simulink model "simulation_quad_modif_nu"  (R2020b)
settings: Solver=VariableStepAuto  StartTime=0.0  StopTime=30  RelTol=1e-3
values from neighbouring files (symbols this model uses):
  controlleur = struct('kap',2.0,                       'kad',4.0,                       'kpp',4.0,                       'kpd',8.0,                       'k_delta',15.0,                       'u_barre',u_barre,                       'M_k',M_k,                       'skew_sym_d_etoile',skew_sym_d_etoile,                       'd_etoile', d_etoile                       )    [generateContolleur.m]    (also in run_quad.m = generateContolleur(drone))
  drone = generatequad()    [run_quad.m]
  f_initial = 1    [run_quad.m]
  initial_state = [p_initial; v_initial; omega_initial; q_initial]    [run_quad.m]
  position_cible = 0.5*[1; 1; 1]    [run_quad.m]
  q_d_initial = ToQuaternion(yaw_d, pitch_d, roll_d)    [run_quad.m]
settings Model: Creator=florian  LastModifiedBy=florian

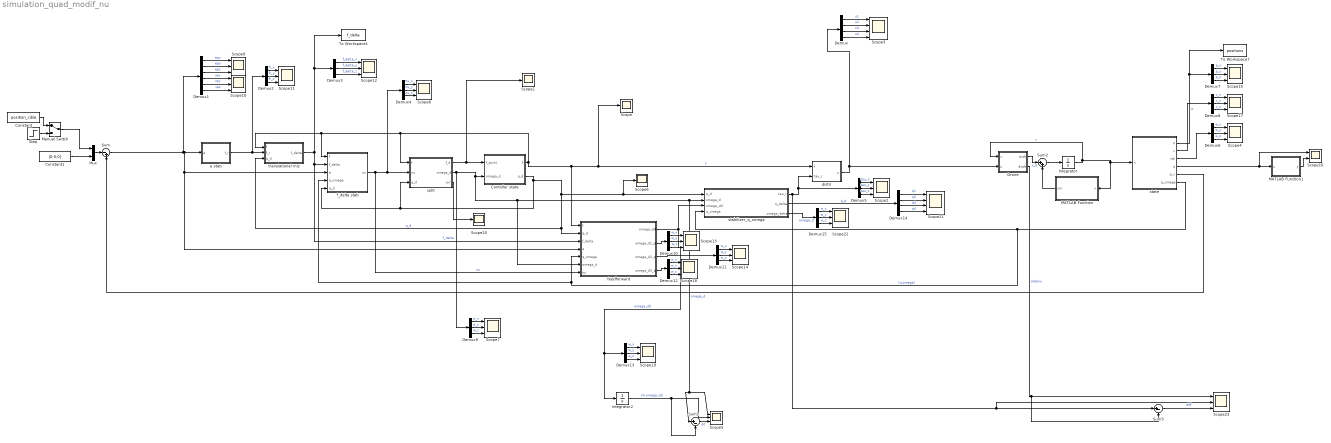
== system simulation_quad_modif_nu ==
  Constant : Constant  Value=position_cible
  Constant1 : Constant  Value=[0;0;0]
  Contoller state : Subsystem
  Demux : Demux
  Demux1 : Demux  Outputs=6
  Demux{2..13,15} (13 alike) : Demux  Outputs=3
  Demux14 : Demux
  Drone : MATLAB Function  TreatAsAtomicUnit=on
  Integrator : Integrator  InitialCondition=initial_state
  Integrator2 : Integrator
  MATLAB Function : MATLAB Function  TreatAsAtomicUnit=on
  MATLAB Function1 : MATLAB Function  TreatAsAtomicUnit=on
  Manual Switch : ManualSwitch
  Mux : Mux  Inputs=2
  Scope{,1,6,20} (4 alike) : Scope
  Scope{2,4..5,7..15,17..19,22..23} (17 alike) : Scope  NumInputPorts=3
  Scope16 : Scope  NumInputPorts=2
  Scope21 : Scope  NumInputPorts=4
  Scope3 : Scope  NumInputPorts=4
  Step : Step  Time=10  Before=position_cible  After=[0;0;0]  SampleTime=0
  Sum : Sum  Inputs=|-+
  Sum1 : Sum  Inputs=|+-
  Sum2 : Sum  Inputs=|++
  Sum3 : Sum  Inputs=|+-
  To Workspace1 : ToWorkspace  VariableName=f_delta  SampleTime=-1
  To Workspace7 : ToWorkspace  VariableName=positions  SampleTime=-1
  distri : MATLAB Function  TreatAsAtomicUnit=on
  e stab : MATLAB Function  TreatAsAtomicUnit=on
  f_delta stab : MATLAB Function  TreatAsAtomicUnit=on
  feedforward : MATLAB Function  TreatAsAtomicUnit=on
  split : MATLAB Function  TreatAsAtomicUnit=on
  stabilizer_q_omega : MATLAB Function  TreatAsAtomicUnit=on
  state : MATLAB Function  TreatAsAtomicUnit=on
  translational mis : MATLAB Function  TreatAsAtomicUnit=on
  wires:
  Integrator/1 -> Drone/1(x), MATLAB Function/1(x), state/1(x)  "x"
  Demux7/2 -> Scope15/2  "p_y"
  state/1(p) -> To Workspace7/1, Demux7/1  "p"
  state/4(q) -> Scope16/1, MATLAB Function1/1(u)
  Demux8/3 -> Scope17/3  "v_z"
  Demux8/1 -> Scope17/1  "v_x"
  MATLAB Function1/1(y) -> Scope16/2
  Demux8/2 -> Scope17/2  "v_y"
  state/2(v) -> Demux8/1
  Demux7/1 -> Scope15/1  "p_x"
  Demux7/3 -> Scope15/3  "p_z"
  Drone/1(dxdt) -> Sum2/1  "x_d"
  Sum2/1 -> Integrator/1
  MATLAB Function/1(cor) -> Sum2/2
  Demux6/2 -> Scope4/2  "w_y"
  Demux6/3 -> Scope4/3  "w_z"
  state/3(wb) -> Demux6/1
  Demux6/1 -> Scope4/1  "w_x"
  Constant1/1 -> Mux/2
  Demux4/2 -> Scope8/2  "nu_y"
  f_delta stab/1(nu) -> feedforward/7(nu), Demux4/1, split/2(nu)  "nu"
  Demux9/1 -> Scope7/1  "w_x"
  Mux/1 -> Sum/1
  split/3(err) -> Scope20/1
  Step/1 -> Manual Switch/2
  Constant/1 -> Manual Switch/1
  Demux11/2 -> Scope14/2  "w_y"
  Contoller state/1(f) -> f_delta stab/1(f), translational mis/1(f), split/1(f), feedforward/1(f), Scope/1, distri/1(f)  "f"
  feedforward/1(omega_dd) -> stabilizer_q_omega/3(omega_dd), Demux13/1, Integrator2/1  "omega_dd"
  Demux13/2 -> Scope19/2  "w_y"
  Demux3/1 -> Scope12/1  "f_delta_x"
  Demux1/4 -> Scope10/1  "vpx"
  Demux/2 -> Scope3/2  "u2"
  Demux9/3 -> Scope7/3  "w_z"
  state/6(q_omega) -> f_delta stab/4(q_omega), feedforward/5(q_omega), stabilizer_q_omega/4(q_omega)  "(q,omega)"
  Demux12/2 -> Scope18/2  "w_y"
  state/5(p_v) -> Sum/2
  Demux3/3 -> Scope12/3  "f_delta_z"
  Manual Switch/1 -> Mux/1
  Demux13/1 -> Scope19/1  "w_x"
  Demux11/3 -> Scope14/3  "w_z"
  Demux/4 -> Scope3/4  "u4"
  Demux2/1 -> Scope11/1  "fr_x"
  Demux13/3 -> Scope19/3  "w_z"
  Demux10/3 -> Scope13/3  "w_z"
  Demux9/2 -> Scope7/2  "w_y"
  Demux5/2 -> Scope2/2  "tau_y"
  e stab/1(f_r) -> Demux2/1, translational mis/2(f_r)
  Demux/1 -> Scope3/1  "u1"
  Demux2/2 -> Scope11/2  "fr_y"
  feedforward/3(omega_d2_p) -> Demux11/1
  Demux15/3 -> Scope22/3  "w_z"
  Demux4/3 -> Scope8/3  "nu_z"
  Demux14/4 -> Scope21/4  "q4"
  split/2(omega_d) -> Demux9/1, feedforward/6(omega_d), Sum1/1, Scope5/1, stabilizer_q_omega/2(omega_d), Contoller state/2(omega_d)  "omega_d"
  Demux4/1 -> Scope8/1  "nu_x"
  Demux14/1 -> Scope21/1  "q1"
  Demux15/2 -> Scope22/2  "w_y"
  Contoller state/2(q_d) -> f_delta stab/5(q_d), split/3(q_d), feedforward/2(q_d), translational mis/3(q_d), Scope6/1, stabilizer_q_omega/1(q_d)  "q_d"
  feedforward/2(omega_d1_p) -> Demux10/1
  Demux15/1 -> Scope22/1  "w_x"
  stabilizer_q_omega/2(q_delta) -> Demux14/1  "q_d"
  Sum1/1 -> Scope5/3  "dif"
  Demux11/1 -> Scope14/1  "w_x"
  Demux12/1 -> Scope18/1  "w_x"
  Demux12/3 -> Scope18/3  "w_z"
  feedforward/4(omega_d3_p) -> Demux12/1
  Demux10/2 -> Scope13/2  "w_y"
  Demux1/2 -> Scope9/2  "epy"
  Demux10/1 -> Scope13/1  "w_x"
  distri/1(u) -> Drone/2(u), Demux/1
  Demux5/1 -> Scope2/1  "tau_x"
  Demux1/6 -> Scope10/3  "vpz"
  split/1(f_d) -> Scope1/1, Contoller state/1(f_point)
  Demux5/3 -> Scope2/3  "tau_z"
  Demux2/3 -> Scope11/3  "fr_z"
  Demux3/2 -> Scope12/2  "f_delta_y"
  stabilizer_q_omega/3(omega_delta) -> Demux15/1  "omega_d"
  Sum/1 -> Demux1/1, feedforward/4(e), f_delta stab/3(e), e stab/1(e)
  translational mis/1(f_delta) -> Demux3/1, To Workspace1/1, feedforward/3(f_delta), f_delta stab/2(f_delta)  "f_delta"
  Demux14/3 -> Scope21/3  "q3"
  Demux1/1 -> Scope9/1  "epx"
  Demux1/3 -> Scope9/3  "epz"
  Demux1/5 -> Scope10/2  "vpy"
  Demux/3 -> Scope3/3  "u3"
  Integrator2/1 -> Sum1/2, Scope5/2  "int omega_dd"
  Demux14/2 -> Scope21/2  "q2"
  Drone/2(dwdt) -> Sum3/2, Scope23/1  "obtenu"
  Sum3/1 -> Scope23/3  "diff"
  stabilizer_q_omega/1(tau_r) -> Scope23/2, Sum3/1, Demux5/1, distri/2(tau_r)

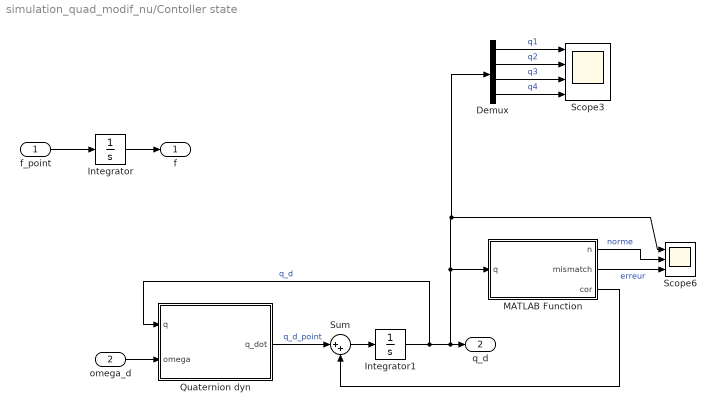
== system simulation_quad_modif_nu/Contoller state ==
  f_point : Inport
  omega_d : Inport  Port=2
  Demux : Demux
  Integrator : Integrator  InitialCondition=f_initial
  Integrator1 : Integrator  InitialCondition=q_d_initial
  MATLAB Function : MATLAB Function  TreatAsAtomicUnit=on
  Quaternion dyn : MATLAB Function  TreatAsAtomicUnit=on
  Scope3 : Scope  NumInputPorts=4
  Scope6 : Scope  NumInputPorts=3
  Sum : Sum  Inputs=|++
  f : Outport
  q_d : Outport  Port=2
  wires:
  Integrator/1 -> f/1
  f_point/1 -> Integrator/1
  Integrator1/1 -> Quaternion dyn/1(q), Demux/1, Scope6/1, MATLAB Function/1(q), q_d/1  "q_d"
  omega_d/1 -> Quaternion dyn/2(omega)
  Quaternion dyn/1(q_dot) -> Sum/1  "q_d_point"
  Sum/1 -> Integrator1/1
  MATLAB Function/3(cor) -> Sum/2
  MATLAB Function/1(n) -> Scope6/2  "norme"
  MATLAB Function/2(mismatch) -> Scope6/3  "erreur"
  Demux/3 -> Scope3/3  "q3"
  Demux/2 -> Scope3/2  "q2"
  Demux/1 -> Scope3/1  "q1"
  Demux/4 -> Scope3/4  "q4"

== matlab function simulation_quad_modif_nu/Contoller state/MATLAB Function ==
  data: n output; q input; mismatch output; cor output
function [n, mismatch, cor] = fcn(q)
%#codegen
n = norm(q);
mismatch = 1-norm(q);
cor = mismatch*q;

== matlab function simulation_quad_modif_nu/MATLAB Function1 ==
  data: u input; y output
function y = fcn(u)
%#codegen

y = norm(u);

== matlab function simulation_quad_modif_nu/Contoller state/Quaternion dyn ==
  data: q input; q_dot output; omega input
function q_dot = q_dyn(q, omega)
%#codegen

eta = q(1);
eps = q(2:4);

A = [-eps';  eta*eye(3)+skew_sym(eps)];
q_dot = 1/2*A*omega;

== matlab function simulation_quad_modif_nu/state ==
  data: x input; p output; v output; wb output; q output; p_v output; q_omega output
function [p, v, wb, q, p_v, q_omega] = demux(x)
%#codegen

p = x(1:3);
v = x(4:6);
wb = x(7:9);
q  = x(10:13);
p_v = x(1:6);
q_omega = [q; wb];

== matlab function simulation_quad_modif_nu/MATLAB Function ==
  data: x input; cor output
function cor  = fcn(x)
%#codegen
q  = x(10:13);
n = norm(q);
mismatch = 1-n;
cor = [0;0;0; 0;0;0; 0;0;0; mismatch*q];

== matlab function simulation_quad_modif_nu/distri ==
  data: f input; u output; tau_r input; controlleur parameter
function u = dist(f,tau_r, controlleur)
%#codegen
u = controlleur.M_k * tau_r + controlleur.u_barre * f;

== matlab function simulation_quad_modif_nu/Drone ==
  data: x input; u input; dxdt output; drone parameter; dwdt output
function [dxdt, dwdt]= drone(x, u, drone)

%% physical constants
% gravity
g = drone.G;
% vehicle mass
m = drone.MASS;
% vehicle inertia matrix
J = drone.INERTIA; % [3x3 real symmetric] in body axis

%% state demultiplexing
% p = x(1:3);
v = x(4:6);
wb = x(7:9);
q  = x(10:13);

Rq = q2dcm(q);

% position
dpdt = v;

% kinematics
dvdt =  -[0;0;g] + (1/m)*Rq*drone.Fb*u; 

%% angular velocity derivative
% kinematics
dwdt = -J\cross(wb, J*wb) + J\(drone.Mb*u);

%% quaternion derivative
eta = q(1);
eps = q(2:4);

dqdt = (1/2)*[-eps'; eta*eye(3) + skew_sym(eps)]*wb;

%% derivative multiplexing
dxdt = [dpdt; dvdt; dwdt; dqdt] ;

== matlab function simulation_quad_modif_nu/stabilizer_q_omega ==
  data: q_d input; omega_d input; omega_dd input; q_omega input; tau_r output; controlleur parameter; drone parameter; q_delta output; omega_delta output
function [tau_r, q_delta, omega_delta]  = stabilizer_q_omega(q_d, omega_d, omega_dd, q_omega, controlleur, drone )

J = drone.INERTIA;

q = q_omega(1:4);
omega = q_omega(5:7);

eta = q(1);
eps = q(2:4);

eta_d = q_d(1);
eps_d = q_d(2:4);

eta_delta = eta_d*eta + eps_d'*eps;
eps_delta = -eta*eps_d + eta_d*eps - skew_sym(eps_d)*eps;

omega_delta = omega - omega_d;

tau_r = - controlleur.kap * eps_delta - controlleur.kad * omega_delta + cross(omega, J* omega) + J*omega_dd;
q_delta = [eta_delta; eps_delta];
end

== matlab function simulation_quad_modif_nu/split ==
  data: f input; nu input; f_d output size=1; q_d input; omega_d output size=3; controlleur parameter; err output
function [f_d, omega_d, err] = split(f, nu, q_d, controlleur)
%#codegen

R_d = q2dcm(q_d);

f_d = (R_d * controlleur.d_etoile)' * nu;
omega_d = 1/f * controlleur.skew_sym_d_etoile * R_d' * nu;

err =  R_d*controlleur.d_etoile*f_d + R_d* skew_sym(omega_d) * controlleur.d_etoile * f - nu;

== matlab function simulation_quad_modif_nu/f_delta stab ==
  data: f input; f_delta input; nu output; e input; q_omega input; q_d input; controlleur parameter; drone parameter
function nu = stab_f_delta(f, f_delta, e, q_omega, q_d, controlleur, drone)
%#codegen
m = drone.MASS;
kpp = controlleur.kpp;
kpd = controlleur.kpd;
k_delta = controlleur.k_delta;

ep = e(1:3);
ev = e(4:6);

q = q_omega(1:4);
% omega = q_omega(5:7);

R = q2dcm(q);
Rd = q2dcm(q_d);

nu = ((kpp * kpd)/m) * ep + (kpd^2/m - kpp) * ev - (kpd/m + k_delta) * f_delta -kpd/m * (R-Rd) * controlleur.d_etoile * f;

== matlab function simulation_quad_modif_nu/translational mis ==
  data: f input; f_r input; f_delta output; q_d input; controlleur parameter
function f_delta = trans_mis(f, f_r,  q_d, controlleur)
%#codegen

f_delta = q2dcm(q_d) * controlleur.d_etoile * f - f_r;

== matlab function simulation_quad_modif_nu/e stab ==
  data: e input; f_r output; drone parameter; controlleur parameter
function f_r = e_stab(e, drone, controlleur)
%#codegen
ep = e(1:3);
ev = e(4:6);

f_r = drone.MASS * [0;0;drone.G] - controlleur.kpp * ep - controlleur.kpd * ev;

== matlab function simulation_quad_modif_nu/feedforward ==
  data: f input; omega_dd output; q_d input; f_delta input; e input; q_omega input; omega_d input; nu input; controlleur parameter; drone parameter; omega_d1_p output; omega_d2_p output; omega_d3_p output
function [omega_dd, omega_d1_p, omega_d2_p, omega_d3_p]  = feedforward(f, q_d, f_delta,e, q_omega,omega_d, nu, controlleur, drone)
%#codegen

d_etoile = controlleur.d_etoile;
kpp = controlleur.kpp;
kpd = controlleur.kpd;
k_delta = controlleur.k_delta;
m = drone.MASS;

ep = e(1:3);
ev = e(4:6);

q = q_omega(1:4);
omega = q_omega(5:7);

R = q2dcm(q);
Rd = q2dcm(q_d);

omega_d1_p = -(1/(f^2)) * skew_sym(d_etoile) * Rd' * nu * ( Rd * d_etoile)' * nu;
omega_d2_p = -(1/(f))* skew_sym(d_etoile) * skew_sym(omega_d) * Rd' * nu;

Gain = (kpd^2/m^2 - kpp/m);

ep_term = - Gain*kpp*ep;
ev_term = (kpp*kpd/m - Gain*kpd)*ev;
f_delta_term = (Gain + (kpd/m + k_delta)*k_delta)*f_delta;
f_term = (Gain*(R-Rd) + kpd/m * (Rd*skew_sym(omega_d) - R*skew_sym(omega)))*d_etoile* f;
nu_term = kpd/m * (Rd-R) * d_etoile * (Rd*d_etoile)'* nu;

omega_d3_p = (1/f) * skew_sym(d_etoile) * Rd'* (ep_term + ev_term + f_delta_term + f_term + nu_term); 

omega_dd = omega_d1_p + omega_d2_p + omega_d3_p ; %
